simulink model "sys_ID"  (R2020b)
settings: Solver=VariableStepAuto  StartTime=0.0  StopTime=10.0  RelTol=1e-3
values from neighbouring files (symbols this model uses):
  den_id = [1 2.004 4.314]    [car_model_parameters.m]
  num_id = 2.398    [car_model_parameters.m]
undefined symbols (not defined in the file or in its folder): den_mylin, num_mylin
settings Model: Creator=arthur  LastModifiedBy=arthur

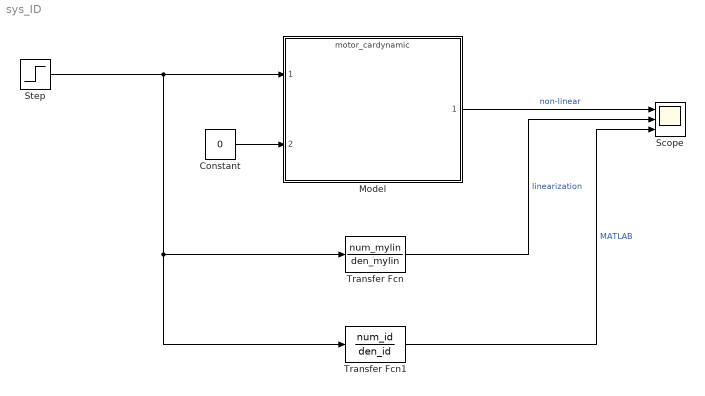
== system sys_ID ==
  Constant : Constant  Value=0
  Model : ModelReference  ModelNameDialog=motor_cardynamic.slx  SimulationMode=Normal  ModelReferenceVersion=1.10
  Scope : Scope  NumInputPorts=3
  Step : Step  SampleTime=0
  Transfer Fcn : TransferFcn  Numerator=num_mylin  Denominator=den_mylin
  Transfer Fcn1 : TransferFcn  Numerator=num_id  Denominator=den_id
  wires:
  Constant/1 -> Model/2
  Step/1 -> Transfer Fcn1/1, Transfer Fcn/1, Model/1
  Model/1 -> Scope/1  "non-linear"
  Transfer Fcn/1 -> Scope/2  "linearization"
  Transfer Fcn1/1 -> Scope/3  "MATLAB"
